simulink model "ysw11_21"  (R2014a)
settings: Solver=ode45  StartTime=0.0  StopTime=10.0  RelTol=1e-3
libraries: commdigbbndam3 x1
settings Model: Creator=ii  LastModifiedBy=ii
settings SolverCC: ZeroCrossAlgorithm=Adaptive
settings DebuggingCC: UnderspecifiedInitializationDetection=Classic

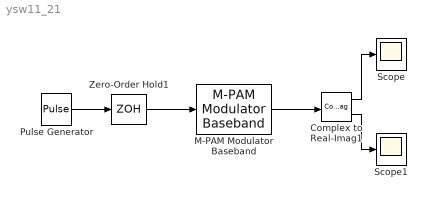
== system ysw11_21 ==
  Complex to Real-Imag1 : ComplexToRealImag
  M-PAM Modulator Baseband : commdigbbndam3/M-PAM Modulator Baseband  M=32  InType=Integer  Enc=Gray  PowType=Min. distance between symbols  MinDist=1  AvgPow=1  PeakPow=1  outDtype=double  outWordLen=16  outUDDataType=sfix(16)  outFracLenMode=Best precision  outFracLen=15
  Pulse Generator : DiscretePulseGenerator  PulseType=Time based  Period=10  PulseWidth=5
  Scope : Scope
  Scope1 : Scope
  Zero-Order Hold1 : ZeroOrderHold
  wires:
  Complex to Real-Imag1/1 -> Scope/1
  Complex to Real-Imag1/2 -> Scope1/1
  M-PAM Modulator Baseband/1 -> Complex to Real-Imag1/1
  Pulse Generator/1 -> Zero-Order Hold1/1
  Zero-Order Hold1/1 -> M-PAM Modulator Baseband/1
